simulink model "matlab"  (R2021b)
settings: Solver=FixedStepAuto  StartTime=0.0  StopTime=inf  RelTol=1e-3
libraries: instrumentlib x1
settings Model: Creator=Juan Ricardo  LastModifiedBy=david
settings SolverCC: AlgebraicLoopSolver=TrustRegion
settings DataIOCC: ReturnWorkspaceOutputs=off
settings DebuggingCC: SFMachineParentedDataDiag=warning  ArithmeticOperatorsInVariantConditions=warning
settings SFSimCC: SimUseLocalCustomCode=off  CustomCodeUndefinedFunction=UseInterfaceOnly
settings RTWCC: RTWUseLocalCustomCode=off

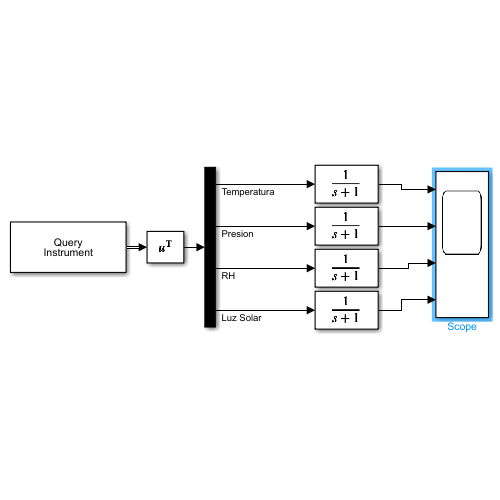
[thumbnail: Simulink's stored preview of the top-level diagram]
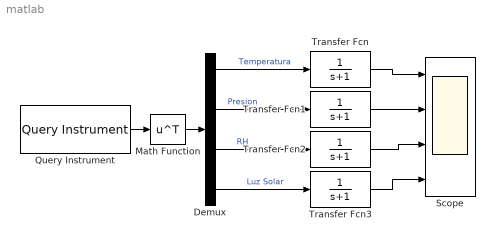
== system matlab ==
  Demux : Demux
  Math Function : Math  Operator=transpose  SignedPower=on  SaturateOnIntegerOverflow=on
  Query Instrument : instrumentlib/Query Instrument  sampleTime=0.05  isWorkspaceObject=off  timeout=10  inputBufferSize=9600  protocol=Serial  serialPort=COM1  baudRate=9600  gpibVendor=Keysight Technologies  boardIndex=0  primaryAddress=1  secondaryAddress=0  visaVendor=Keysight  visaSerialPort=0  chassisIndex=0  logicalAddress=0  tcpRemoteHost='127.0.0.1'  tcpRemotePort=4500  udpRemoteHost='127.0.0.1'  udpRemotePort=9090  visaTCPBoardIndex=0  visaTCPRemoteHost='127.0.0.1'  usbBoardIndex=0  usbManufID=0  usbModelCode=0  usbSerialNumber=0  initAction=None  initCommand='DATA:SOURCE CH1'  initFunction=get  queryCommand=''  responseFormat=ASCII  asciiFormatting='S%d,%d,%d,%d'  precision=8-bit integer  byteOrder=Little endian  valuesToRead=1  removeBytes=off  afterOutputAction=Repeat query for new data  enableFrames=on  frameSize=4
      settings: SourceProductBaseCode=IC
  Scope : Scope  NumInputPorts=4
  Transfer Fcn{,1..3} (4 alike) : TransferFcn  Denominator=[1 1]
  wires:
  Query Instrument/1 -> Math Function/1
  Math Function/1 -> Demux/1
  Demux/1 -> Transfer Fcn/1  "Temperatura"
  Transfer Fcn/1 -> Scope/1
  Demux/4 -> Transfer Fcn3/1  "Luz Solar"
  Transfer Fcn3/1 -> Scope/4
  Demux/2 -> Transfer Fcn1/1  "Presion"
  Demux/3 -> Transfer Fcn2/1  "RH"
  Transfer Fcn1/1 -> Scope/2
  Transfer Fcn2/1 -> Scope/3
